simulink model "Cowley_315Week8HWSim"  (R2020b)
settings: Solver=VariableStepAuto  StartTime=0.0  StopTime=10.0  RelTol=1e-3
values from neighbouring files (symbols this model uses):
  c = 0    [Cowley_315Exam2TakeHome.m]    (also in Cowley_315Week8HW_Prob1.m = 20000; Cowley_315Week8HW_Prob2.m = 17.07; Cowley_FinalTakeHome1.m = [c1 c2]; ForceInputResponse.m = 19)
  k = 1    [Cowley_315Exam2TakeHome.m]    (also in Cowley_315Week4HW_Problem3.m = 100; Cowley_315Week8HW_Prob1.m = 400000; Cowley_315Week8HW_Prob2.m = 500; Cowley_FinalTakeHome1.m = [k1 k2])
  m = 1    [Cowley_315Exam2TakeHome.m]    (also in Cowley_315Week4HW_Problem3.m = 10; Cowley_315Week8HW_Prob1.m = 1007; Cowley_315Week8HW_Prob2.m = 0.4; Cowley_FinalTakeHome1.m = [m1 m2])
  v0 = 0    [Cowley_315Exam2TakeHome.m]    (also in Cowley_315Week13HW_Problem1.m = [0;0]; Cowley_315Week13HW_Problem2.m = [0;0;1]; Cowley_315Week13_Problem3.m = [1 0]; Cowley_315Week4HW_Problem3.m = 10)
  wb = 5.8    [Cowley_315Week8HW_Prob1.m]
  x0 = 0    [Cowley_315Exam2TakeHome.m]    (also in Cowley_315Week13HW_Problem1.m = [0.1;1]; Cowley_315Week13HW_Problem2.m = zeros(3,1); Cowley_315Week13_Problem3.m = [0 0.1]; Cowley_315Week4HW_Problem3.m)
  Y = 0.01    [Cowley_315Week8HW_Prob1.m]
settings Model: Creator=mattcowley  LastModifiedBy=mattcowley

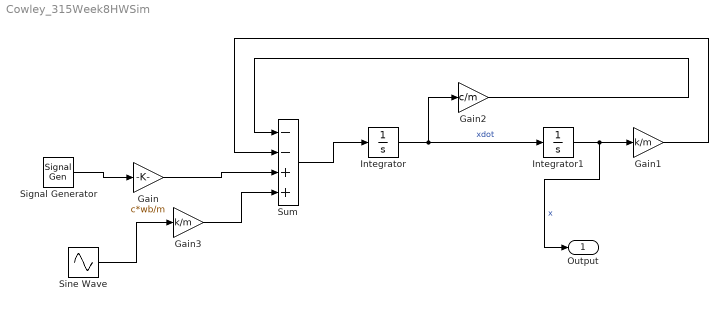
== system Cowley_315Week8HWSim ==
  Gain : Gain  Gain=c*wb/m
  Gain1 : Gain  Gain=k/m
  Gain2 : Gain  Gain=c/m
  Gain3 : Gain  Gain=k/m
  Integrator : Integrator  InitialCondition=v0
  Integrator1 : Integrator  InitialCondition=x0
  Signal Generator : SignalGenerator  Amplitude=Y  Frequency=wb  Units=rad/sec
  Sine Wave : Sin  Amplitude=Y  Frequency=wb  Phase=pi/2  SampleTime=0
  Sum : Sum  Inputs=--++
  Output : Outport  SignalName=x
  wires:
  Sum/1 -> Integrator/1
  Integrator/1 -> Gain2/1, Integrator1/1  "xdot"
  Integrator1/1 -> Output/1, Gain1/1  "x"
  Gain2/1 -> Sum/1
  Gain1/1 -> Sum/2
  Signal Generator/1 -> Gain/1
  Gain/1 -> Sum/3
  Gain3/1 -> Sum/4
  Sine Wave/1 -> Gain3/1
